simulink model "MotorCtrl_FOC_Math"  (R2025b)
settings: Solver=FixedStepDiscrete  StartTime=0.0  StopTime=5  FixedStep=MC_Sim_BaseStep  RelTol=1e-3  EnableMultiTasking=on
values from neighbouring files (symbols this model uses):
  MC_ADC_BitNum = 0.0    [MotorControlDataDictionary_Math.sldd]
  MC_ADC_Offset = 0.0    [MotorControlDataDictionary_Math.sldd]
  MC_ADC_VRef = 1.0    [MotorControlDataDictionary_Math.sldd]
  MC_CSA_Gain = 1.0    [MotorControlDataDictionary_Math.sldd]
  MC_MOS_DeadTime = 1.3E-6    [MotorControlDataDictionary_Math.sldd]
  MC_Motor_Mechinal_Damp = 1.0E-5    [MotorControlDataDictionary_Math.sldd]
  MC_Motor_Mechinal_Fric = 0.0    [MotorControlDataDictionary_Math.sldd]
  MC_Motor_Mechinal_Inertia = 0.0103    [MotorControlDataDictionary_Math.sldd]
  MC_Motor_Phi = 0.0059190254913385806    [MotorControlDataDictionary_Math.sldd]
  MC_Motor_Rotor_Pn = 4.0    [MotorControlDataDictionary_Math.sldd]
  MC_Motor_Stator_Ld = 5.6345E-5    [MotorControlDataDictionary_Math.sldd]
  MC_Motor_Stator_Lq = 5.6345E-5    [MotorControlDataDictionary_Math.sldd]
  MC_Motor_Stator_Rs = 0.0286    [MotorControlDataDictionary_Math.sldd]
  MC_Param_CurrentPI_Ki = 0.0089705790612839825    [MotorControlDataDictionary_Math.sldd]
  MC_Param_CurrentPI_Kp = 0.283220860906427    [MotorControlDataDictionary_Math.sldd]
  MC_Param_CurrentPI_UdInteMax = 7.794228634059948    [MotorControlDataDictionary_Math.sldd]
  MC_Param_CurrentPI_UdInteMin = -7.794228634059948    [MotorControlDataDictionary_Math.sldd]
  MC_Param_CurrentPI_UdMax = 7.794228634059948    [MotorControlDataDictionary_Math.sldd]
  MC_Param_CurrentPI_UdMin = -7.794228634059948    [MotorControlDataDictionary_Math.sldd]
  MC_Param_CurrentPI_UqInteMax = 7.794228634059948    [MotorControlDataDictionary_Math.sldd]
  MC_Param_CurrentPI_UqInteMin = -7.794228634059948    [MotorControlDataDictionary_Math.sldd]
  MC_Param_CurrentPI_UqMax = 7.794228634059948    [MotorControlDataDictionary_Math.sldd]
  MC_Param_CurrentPI_UqMin = -7.794228634059948    [MotorControlDataDictionary_Math.sldd]
  MC_Param_Flux_Gamma = 750000.0    [MotorControlDataDictionary_Math.sldd]
  MC_Param_Flux_Lalpha = 5.6345E-5    [MotorControlDataDictionary_Math.sldd]
  MC_Param_Flux_Lbeta = 5.6345E-5    [MotorControlDataDictionary_Math.sldd]
  MC_Param_Flux_Ralpha = 0.0286    [MotorControlDataDictionary_Math.sldd]
  MC_Param_Flux_Rbeta = 0.0286    [MotorControlDataDictionary_Math.sldd]
  MC_Param_Luen_BEMFalpha = -17747.803709290976    [MotorControlDataDictionary_Math.sldd]
  MC_Param_Luen_BEMFbeta = -17747.803709290976    [MotorControlDataDictionary_Math.sldd]
  MC_Param_Luen_BEMFErr = 10.0    [MotorControlDataDictionary_Math.sldd]
  MC_Param_Luen_Currentalpha = -507.58718608572195    [MotorControlDataDictionary_Math.sldd]
  MC_Param_Luen_Currentbeta = -507.58718608572195    [MotorControlDataDictionary_Math.sldd]
  MC_Param_Luen_CurrentErr = 400.0    [MotorControlDataDictionary_Math.sldd]
  MC_Param_Luen_PLL_Ki = 0.24634532585119037    [MotorControlDataDictionary_Math.sldd]
  MC_Param_Luen_PLL_Kp = 125.66370614359172    [MotorControlDataDictionary_Math.sldd]
  MC_Param_Luen_Voltagealpha = 17747.803709290976    [MotorControlDataDictionary_Math.sldd]
  MC_Param_Luen_Voltagebeta = 17747.803709290976    [MotorControlDataDictionary_Math.sldd]
  MC_Param_PhasetoReal = 500.0    [MotorControlDataDictionary_Math.sldd]
  MC_Param_SMO_CoffA = 0.968326559588251    [MotorControlDataDictionary_Math.sldd]
  MC_Param_SMO_CoffB = 1.1074629514597569    [MotorControlDataDictionary_Math.sldd]
  MC_Param_SpeedCtrl_IdMax = 60.0    [MotorControlDataDictionary_Math.sldd]
  MC_Param_SpeedCtrl_IdMin = -60.0    [MotorControlDataDictionary_Math.sldd]
  MC_Param_SpeedCtrl_IqMax = 60.0    [MotorControlDataDictionary_Math.sldd]
  MC_Param_SpeedCtrl_IqMin = -60.0    [MotorControlDataDictionary_Math.sldd]
  MC_Param_SpeedPI_Ki = 0.57157085739428382    [MotorControlDataDictionary_Math.sldd]
  MC_Param_SpeedPI_Kp = 9.1114109857344836    [MotorControlDataDictionary_Math.sldd]
  MC_Param_SpeedtoTheta = 6.24E-5    [MotorControlDataDictionary_Math.sldd]
  MC_Param_SVPWM_DutyMax = 0.98    [MotorControlDataDictionary_Math.sldd]
  MC_Param_SVPWM_DutyMin = 0.02    [MotorControlDataDictionary_Math.sldd]
  MC_Param_SVPWM_SampleOffset1 = 0.02    [MotorControlDataDictionary_Math.sldd]
  MC_Param_SVPWM_SampleOffset2 = 0.015    [MotorControlDataDictionary_Math.sldd]
  MC_Param_SVPWM_SampleValid = 0.0096153846153846159    [MotorControlDataDictionary_Math.sldd]
  MC_Param_Zero = 0.0    [MotorControlDataDictionary_Math.sldd]
  MC_Sample_CurrentNoise = 1.0E-15    [MotorControlDataDictionary_Math.sldd]
  MC_Sample_Rs = 0.002    [MotorControlDataDictionary_Math.sldd]
  MC_Sample_VbusNoise = 1.0E-15    [MotorControlDataDictionary_Math.sldd]
  MC_Sim_BaseStep = 2.08E-8    [MotorControlDataDictionary_Math.sldd]
  MC_Sim_HFTStep = 6.24E-5    [MotorControlDataDictionary_Math.sldd]
  MC_Sim_MFTStep = 0.0019968    [MotorControlDataDictionary_Math.sldd]
libraries: simulink x28, nesl_utility x19, fl_lib x14, ee_lib x13, autolibpmsminterior x2, autolibinverter x1
(part 4 of 8)

== system MotorCtrl_FOC_Math/MFTask/adrcofSpeed ==
  SpeedTarget : Inport
  SpeedReal : Inport  Port=2
  Constant : Constant  Value=0  OutDataTypeStr=single
  Delay One Step : Delay  DelayLength=1  InitialCondition=MC_Param_Zero
  ESO : Subsystem
  LESO : Subsystem  VariantControl=ESO
  NLSEF : Subsystem
  Tracking-Differentiator : Subsystem  Commented=on
  IdRef : Outport
  IqRef : Outport  Port=2
  wires:
  SpeedTarget/1 -> NLSEF/1(" SpeedRef"), Tracking-Differentiator/1(Ref_In)
  NLSEF/1(IqRef) -> IqRef/1, Delay One Step/1
  Tracking-Differentiator/1(SpeedTarget_TD) -> ?
  Delay One Step/1 -> ESO/2(u)
  ESO/1(z1) -> NLSEF/2(" z")
  ESO/2(z2) -> NLSEF/3(" d")
  Constant/1 -> IdRef/1
  SpeedReal/1 -> ESO/1(SpeedReal)

== system MotorCtrl_FOC_Math/MFTask/getCurrentLimit ==
  IdRef : Inport
  IqRef : Inport  Port=2
  Saturation : Saturate  UpperLimit=MC_Param_SpeedCtrl_IqMax  LowerLimit=MC_Param_SpeedCtrl_IqMin
  Saturation1 : Saturate  UpperLimit=MC_Param_SpeedCtrl_IdMax  LowerLimit=MC_Param_SpeedCtrl_IdMin
  Signal Copy : SignalConversion  OverrideOpt=off
  Signal Copy1 : SignalConversion  OverrideOpt=off
  IdRefLimit : Outport
  IqRefLimit : Outport  Port=2
  wires:
  IqRef/1 -> Saturation/1
  IdRef/1 -> Saturation1/1
  Signal Copy/1 -> IdRefLimit/1  "IdRefLimit"
  Signal Copy1/1 -> IqRefLimit/1  "IqRefLimit"
  Saturation/1 -> Signal Copy1/1
  Saturation1/1 -> Signal Copy/1

== system MotorCtrl_FOC_Math/MFTask/piofSpeed ==
  SpeedTarget : Inport
  SpeedReal : Inport  Port=2
  Abs : Abs  SaturateOnIntegerOverflow=off
  Add : Sum
  Add1 : Sum
  Compare To Constant : simulink/Logic and Bit Operations/Compare To Constant  relop=>  const=0.01  OutDataTypeStr=boolean
  Constant : Constant  Value=0  OutDataTypeStr=single
  Constant1 : Constant  Value=0  OutDataTypeStr=single
  Delay One Step : Delay  DelayLength=1
  Gain : Gain  Gain=MC_Param_SpeedPI_Kp
  Gain1 : Gain  Gain=MC_Param_SpeedPI_Ki
  Saturation : Saturate  UpperLimit=50  LowerLimit=-50
  Saturation1 : Saturate  UpperLimit=50  LowerLimit=-50
  Subtract : Sum  Inputs=+-
  Switch : Switch  Criteria=u2 > Threshold  SaturateOnIntegerOverflow=off  InputSameDT=off
  IdRef : Outport
  IqRef : Outport  Port=2
  wires:
  Add/1 -> Saturation/1, Delay One Step/1
  Subtract/1 -> Switch/1, Abs/1, Gain/1
  Gain1/1 -> Add/1
  Saturation/1 -> Add1/2
  Delay One Step/1 -> Add/2
  Gain/1 -> Add1/1
  Compare To Constant/1 -> Switch/2
  Add1/1 -> Saturation1/1
  Abs/1 -> Compare To Constant/1
  Constant/1 -> Switch/3
  SpeedReal/1 -> Subtract/2
  SpeedTarget/1 -> Subtract/1
  Switch/1 -> Gain1/1
  Constant1/1 -> IdRef/1  "IdRef"
  Saturation1/1 -> IqRef/1  "IqRef"

== system MotorCtrl_FOC_Math/MFTask/smcofSpeed ==
  note: 滑模控制：
      | 构建状态变量
  SpeedTarget : Inport
  SpeedReal : Inport  Port=2
  Add : Sum
  Add1 : Sum
  Add2 : Sum
  Constant : Constant  Value=0  OutDataTypeStr=single
  Delay One Step : Delay  DelayLength=1
  Delay One Step1 : Delay  DelayLength=1
  Gain : Gain  Gain=1/MC_Sim_MFTStep
  Gain1 : Gain  Gain=200
  Gain2 : Gain  Gain=50
  Gain3 : Gain  Gain=MC_Sim_MFTStep*1*MC_Motor_Mechinal_Inertia/(3*MC_Motor_Phi*MC_Motor_Rotor_Pn)
  Saturation : Saturate  UpperLimit=2  LowerLimit=-2
  Subtract : Sum  Inputs=+-
  Subtract1 : Sum  Inputs=+-
  IdRef : Outport
  IqRef : Outport  Port=2
  wires:
  SpeedTarget/1 -> Subtract/1
  SpeedReal/1 -> Subtract/2
  Subtract/1 -> Delay One Step/1, Subtract1/1, Add/1  "E1"
  Delay One Step/1 -> Subtract1/2
  Subtract1/1 -> Gain/1
  Gain/1 -> Add/2, Gain2/1  "E2"
  Add/1 -> Saturation/1  "S"
  Saturation/1 -> Gain1/1  "sign(S)"
  Gain1/1 -> Add1/1
  Gain2/1 -> Add1/2
  Add1/1 -> Gain3/1  "IqRef_dot"
  Gain3/1 -> Add2/1
  Add2/1 -> IqRef/1, Delay One Step1/1  "IqRef"
  Delay One Step1/1 -> Add2/2
  Constant/1 -> IdRef/1  "IdRef"

== system MotorCtrl_FOC_Math/Tracking-Differentiator/fastFunc1_TD ==
  Ref_In : Inport
  X1 : Inport  Port=2
  X2 : Inport  Port=3
  Abs1 : Abs  SaturateOnIntegerOverflow=off
  Add : Sum
  Add1 : Sum
  Add2 : Sum
  Constant : Constant  Value=0.01  OutDataTypeStr=single
  Gain : Gain  Gain=MC_Sim_MFTStep  ParamDataTypeStr=single  OutDataTypeStr=single  RndMeth=Simplest
  Gain1 : Gain  Gain=MC_Sim_MFTStep  ParamDataTypeStr=single  OutDataTypeStr=single  RndMeth=Simplest
  Gain2 : Gain  Gain=MC_Sim_MFTStep  ParamDataTypeStr=single  OutDataTypeStr=single  RndMeth=Simplest
  Gain3 : Gain  Gain=8  ParamDataTypeStr=single  OutDataTypeStr=single  RndMeth=Simplest
  Gain4 : Gain  Gain=1/2  ParamDataTypeStr=single  OutDataTypeStr=single  RndMeth=Simplest
  Gain5 : Gain  Gain=1/MC_Sim_MFTStep  ParamDataTypeStr=single  OutDataTypeStr=single  RndMeth=Simplest
  Gain6 : Gain  Commented=on
  Gain7 : Gain  Gain=1/MC_Sim_MFTStep  ParamDataTypeStr=single  OutDataTypeStr=single  RndMeth=Simplest
  Gain8 : Gain  Gain=-1  ParamDataTypeStr=single  OutDataTypeStr=single  RndMeth=Simplest
  Product : Product  OutDataTypeStr=single  RndMeth=Simplest
  Product1 : Product
  Product2 : Product  Commented=on
  Relational Operator : RelationalOperator  Operator=>  OutDataTypeStr=boolean  RndMeth=Simplest  InputSameDT=off
  Relational Operator1 : RelationalOperator  Operator=<=  OutDataTypeStr=boolean  RndMeth=Simplest  InputSameDT=off
  Sign : Signum
  Sign1 : Signum  Commented=on
  Sqrt : Sqrt
  Square : Math  Operator=square
  Subtract : Sum  Inputs=+-
  Subtract1 : Sum  Inputs=+-
  Switch : Switch  Criteria=u2 > Threshold  OutDataTypeStr=single  RndMeth=Simplest  SaturateOnIntegerOverflow=off  InputSameDT=off
  Switch1 : Switch  Criteria=u2 > Threshold  OutDataTypeStr=single  RndMeth=Simplest  SaturateOnIntegerOverflow=off  InputSameDT=off
  Ref_TD : Outport
  wires:
  X2/1 -> [x2]
  Ref_In/1 -> [Ref_In]
  X1/1 -> [x1]
  [x2] -> Gain/1
  Gain/1 -> Add/2
  [e] -> Add/1
  Add/1 -> [y]  "y"
  Subtract/1 -> [e]  "e"
  Constant/1 -> Gain3/1, Product1/2, Gain1/1  "r"
  Gain1/1 -> Gain2/1, [d]  "d"
  Gain2/1 -> [d0]  "d0"
  [y] -> Relational Operator/1, Sign1/1, Product/2
  Gain3/1 -> Product/1
  [d] -> Subtract1/2, Square/1
  Product/1 -> Add1/1
  Square/1 -> Add1/2
  Add1/1 -> Sqrt/1
  [d0] -> Relational Operator/2
  Relational Operator/1 -> Switch/2  "y_d0_Comp"
  Switch/1 -> Add2/1
  [x2] -> Add2/2
  [a0] -> Subtract1/1
  Subtract1/1 -> Gain4/1
  Gain4/1 -> Switch/1  "(a0-d)/2"
  [y] -> Gain5/1
  Gain5/1 -> Switch/3  "y/h"
  Add2/1 -> [a]  "a"
  Abs1/1 -> Relational Operator1/1
  [d] -> Relational Operator1/2
  Relational Operator1/1 -> Switch1/2  "a_d_Comp"
  Switch1/1 -> Gain8/1  "Ref_TD"
  [a] -> Gain7/1, Sign/1, Abs1/1
  Gain7/1 -> Switch1/1  "ra/d"
  Sign/1 -> Product1/1
  Product1/1 -> Switch1/3  "rsign(a)"
  Gain8/1 -> Ref_TD/1  "N_Ref_TD"
  [x1] -> Subtract/1
  [Ref_In] -> Subtract/2
  Sign1/1 -> Gain6/1
  Sqrt/1 -> [a0], Product2/1  "a0"
  Gain6/1 -> Product2/2

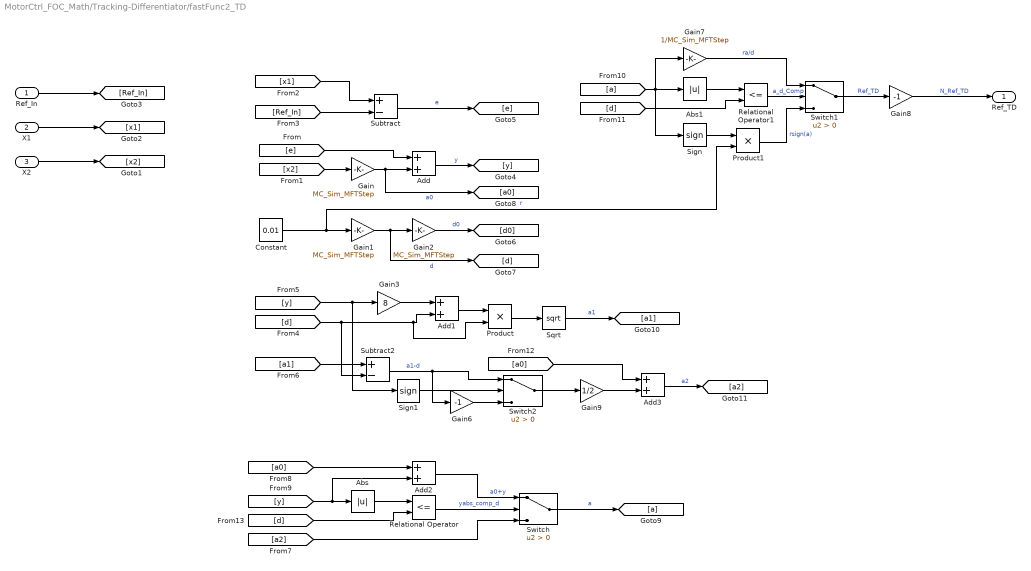
== system MotorCtrl_FOC_Math/Tracking-Differentiator/fastFunc2_TD ==
  Ref_In : Inport
  X1 : Inport  Port=2
  X2 : Inport  Port=3
  Abs : Abs  SaturateOnIntegerOverflow=off
  Abs1 : Abs  SaturateOnIntegerOverflow=off
  Add{,1..3} (4 alike) : Sum
  Constant : Constant  Value=0.01  OutDataTypeStr=single
  Gain : Gain  Gain=MC_Sim_MFTStep  ParamDataTypeStr=single  OutDataTypeStr=single  RndMeth=Simplest
  Gain1 : Gain  Gain=MC_Sim_MFTStep  ParamDataTypeStr=single  OutDataTypeStr=single  RndMeth=Simplest
  Gain2 : Gain  Gain=MC_Sim_MFTStep  ParamDataTypeStr=single  OutDataTypeStr=single  RndMeth=Simplest
  Gain3 : Gain  Gain=8
  Gain6 : Gain  Gain=-1  ParamDataTypeStr=single  OutDataTypeStr=single  RndMeth=Simplest
  Gain7 : Gain  Gain=1/MC_Sim_MFTStep  ParamDataTypeStr=single  OutDataTypeStr=single  RndMeth=Simplest
  Gain8 : Gain  Gain=-1  ParamDataTypeStr=single  OutDataTypeStr=single  RndMeth=Simplest
  Gain9 : Gain  Gain=1/2  ParamDataTypeStr=single  OutDataTypeStr=single  RndMeth=Simplest
  Product : Product
  Product1 : Product
  Relational Operator : RelationalOperator  Operator=<=  OutDataTypeStr=boolean  RndMeth=Simplest  InputSameDT=off
  Relational Operator1 : RelationalOperator  Operator=<=  OutDataTypeStr=boolean  RndMeth=Simplest  InputSameDT=off
  Sign : Signum
  Sign1 : Signum
  Sqrt : Sqrt
  Subtract : Sum  Inputs=+-
  Subtract2 : Sum  Inputs=+-  OutDataTypeStr=single  RndMeth=Simplest
  Switch : Switch  Criteria=u2 > Threshold  OutDataTypeStr=single  RndMeth=Simplest  SaturateOnIntegerOverflow=off  InputSameDT=off
  Switch1 : Switch  Criteria=u2 > Threshold  OutDataTypeStr=single  RndMeth=Simplest  SaturateOnIntegerOverflow=off  InputSameDT=off
  Switch2 : Switch  Criteria=u2 > Threshold  OutDataTypeStr=single  RndMeth=Simplest  SaturateOnIntegerOverflow=off  InputSameDT=off
  Ref_TD : Outport
  wires:
  [Ref_In] -> Subtract/2
  [x1] -> Subtract/1
  Gain8/1 -> Ref_TD/1  "N_Ref_TD"
  Product1/1 -> Switch1/3  "rsign(a)"
  Sign/1 -> Product1/1
  Gain7/1 -> Switch1/1  "ra/d"
  [a] -> Abs1/1, Sign/1, Gain7/1
  Switch1/1 -> Gain8/1  "Ref_TD"
  Relational Operator1/1 -> Switch1/2  "a_d_Comp"
  [d] -> Relational Operator1/2
  Abs1/1 -> Relational Operator1/1
  Gain3/1 -> Add1/1
  [d] -> Subtract2/2, Add1/2, Product/2
  Gain2/1 -> [d0]  "d0"
  Gain1/1 -> [d], Gain2/1  "d"
  Constant/1 -> Product1/2, Gain1/1  "r"
  Subtract/1 -> [e]  "e"
  Add/1 -> [y]  "y"
  [e] -> Add/1
  Gain/1 -> [a0], Add/2  "a0"
  [x2] -> Gain/1
  X1/1 -> [x1]
  Ref_In/1 -> [Ref_In]
  X2/1 -> [x2]
  [y] -> Sign1/1, Gain3/1
  Add1/1 -> Product/1
  Product/1 -> Sqrt/1
  Sqrt/1 -> [a1]  "a1"
  Sign1/1 -> Switch2/2
  [a1] -> Subtract2/1
  Subtract2/1 -> Gain6/1, Switch2/1  "a1-d"
  Gain6/1 -> Switch2/3
  Switch2/1 -> Gain9/1
  Gain9/1 -> Add3/2
  [a0] -> Add3/1
  Add3/1 -> [a2]  "a2"
  [y] -> Add2/2, Abs/1
  Abs/1 -> Relational Operator/1
  Relational Operator/1 -> Switch/2  "yabs_comp_d"
  [d] -> Relational Operator/2
  [a0] -> Add2/1
  Add2/1 -> Switch/1  "a0+y"
  [a2] -> Switch/3
  Switch/1 -> [a]  "a"

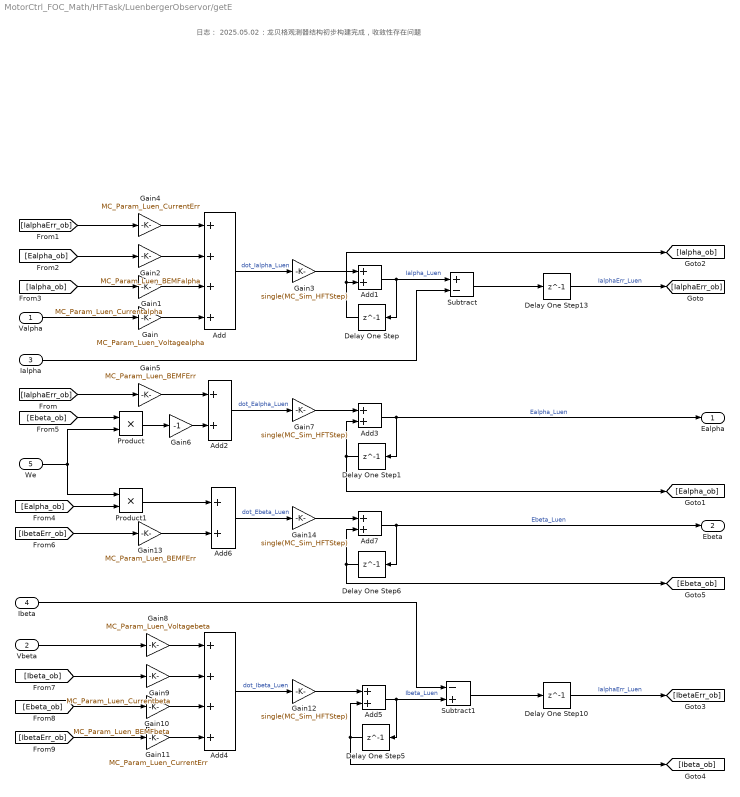
== system MotorCtrl_FOC_Math/HFTask/LuenbergerObservor/getE ==
  note: 日志：
      | 2025.05.02：龙贝格观测器结构初步构建完成，收敛性存在问题
  Valpha : Inport
  Vbeta : Inport  Port=2
  Ialpha : Inport  Port=3
  Ibeta : Inport  Port=4
  We : Inport  Port=5
  Add : Sum  Inputs=++++
  Add{1..3,5..7} (6 alike) : Sum
  Add4 : Sum  Inputs=++++
  Delay One Step{,1,5..6,10,13} (6 alike) : Delay  DelayLength=1
  Gain : Gain  Gain=MC_Param_Luen_Voltagealpha
  Gain1 : Gain  Gain=MC_Param_Luen_Currentalpha
  Gain10 : Gain  Gain=MC_Param_Luen_BEMFbeta
  Gain11 : Gain  Gain=MC_Param_Luen_CurrentErr
  Gain{3,7,12,14} (4 alike) : Gain  Gain=single(MC_Sim_HFTStep)
  Gain13 : Gain  Gain=MC_Param_Luen_BEMFErr
  Gain2 : Gain  Gain=MC_Param_Luen_BEMFalpha
  Gain4 : Gain  Gain=MC_Param_Luen_CurrentErr
  Gain5 : Gain  Gain=MC_Param_Luen_BEMFErr
  Gain6 : Gain  Gain=-1
  Gain8 : Gain  Gain=MC_Param_Luen_Voltagebeta
  Gain9 : Gain  Gain=MC_Param_Luen_Currentbeta
  Product : Product
  Product1 : Product
  Subtract : Sum  Inputs=+-
  Subtract1 : Sum  Inputs=-+
  Ealpha : Outport
  Ebeta : Outport  Port=2
  wires:
  Valpha/1 -> Gain/1
  Add/1 -> Gain3/1  "dot_Ialpha_Luen"
  Gain2/1 -> Add/2
  Gain1/1 -> Add/3
  Gain/1 -> Add/4
  Gain4/1 -> Add/1
  Gain3/1 -> Add1/1
  Add1/1 -> Subtract/1, Delay One Step/1  "Ialpha_Luen"
  Delay One Step/1 -> [Ialpha_ob], Add1/2
  Ialpha/1 -> Subtract/2
  Subtract/1 -> Delay One Step13/1
  [IalphaErr_ob] -> Gain5/1
  Gain5/1 -> Add2/1
  Gain6/1 -> Add2/2
  Add2/1 -> Gain7/1  "dot_Ealpha_Luen"
  Delay One Step1/1 -> Add3/2, [Ealpha_ob]
  Add3/1 -> Ealpha/1, Delay One Step1/1  "Ealpha_Luen"
  Gain7/1 -> Add3/1
  Product/1 -> Gain6/1
  We/1 -> Product/2, Product1/1
  Vbeta/1 -> Gain8/1
  Gain8/1 -> Add4/1
  Gain9/1 -> Add4/2
  Gain10/1 -> Add4/3
  Gain11/1 -> Add4/4
  [IalphaErr_ob] -> Gain4/1
  [Ealpha_ob] -> Gain2/1
  [Ialpha_ob] -> Gain1/1
  Add4/1 -> Gain12/1  "dot_Ibeta_Luen"
  Delay One Step5/1 -> Add5/2, [Ibeta_ob]
  Add5/1 -> Subtract1/2, Delay One Step5/1  "Ibeta_Luen"
  Gain12/1 -> Add5/1
  Ibeta/1 -> Subtract1/1
  Subtract1/1 -> Delay One Step10/1
  Add6/1 -> Gain14/1  "dot_Ebeta_Luen"
  Gain13/1 -> Add6/2
  Product1/1 -> Add6/1
  Gain14/1 -> Add7/1
  Add7/1 -> Ebeta/1, Delay One Step6/1  "Ebeta_Luen"
  Delay One Step6/1 -> Add7/2, [Ebeta_ob]
  [Ealpha_ob] -> Product1/2
  [Ebeta_ob] -> Product/1
  [IbetaErr_ob] -> Gain13/1
  [Ibeta_ob] -> Gain9/1
  [IbetaErr_ob] -> Gain11/1
  [Ebeta_ob] -> Gain10/1
  Delay One Step13/1 -> [IalphaErr_ob]  "IalphaErr_Luen"
  Delay One Step10/1 -> [IbetaErr_ob]  "IalphaErr_Luen"

== system MotorCtrl_FOC_Math/HFTask/LuenbergerObservor/getSpeedandTheta ==
  note: 日志：
      | 2025.03.19：反电势正负号识别错误，改正后可以使用
  Ealpha : Inport
  Ebeta : Inport  Port=2
  Add : Sum
  Add1 : Sum
  Add2 : Sum
  Constant : Constant  Value=2*pi  OutDataTypeStr=single
  Delay One Step : Delay  DelayLength=1
  Delay One Step2 : Delay  DelayLength=1
  Gain1 : Gain  Gain=MC_Param_Luen_PLL_Kp
  Gain2 : Gain  Gain=MC_Param_Luen_PLL_Ki
  Gain3 : Gain  Gain=MC_Param_SpeedtoTheta
  Gain5 : Gain  Gain=30/(pi*MC_Motor_Rotor_Pn)  OutDataTypeStr=single  RndMeth=Simplest
  Mod : Math  Operator=mod
  Product : Product
  Product1 : Product
  Sin : Trigonometry  OutputSignalType=real
  Sin1 : Trigonometry  Operator=cos  OutputSignalType=real
  Subtract : Sum  Inputs=+-
  Speed : Outport
  Theta : Outport  Port=2
  We : Outport  Port=3
  wires:
  Gain5/1 -> Speed/1  "SpeedLuen_RPM"
  Product1/1 -> Subtract/2  "LuenCos"
  Product/1 -> Subtract/1  "LuenSin"
  [Theta_Last] -> Sin/1, Sin1/1
  Add1/1 -> We/1, Gain3/1, Gain5/1  "WeLuen"
  Mod/1 -> Delay One Step2/1, Theta/1  "ThetaLuen"
  Delay One Step2/1 -> [Theta_Last], Add2/2
  Constant/1 -> Mod/2
  Add2/1 -> Mod/1
  Gain3/1 -> Add2/1
  Subtract/1 -> Gain1/1, Gain2/1  "LuenErr"
  Gain1/1 -> Add1/1
  Delay One Step/1 -> Add/2
  Add/1 -> Add1/2, Delay One Step/1
  Gain2/1 -> Add/1
  Sin/1 -> Product1/2
  Sin1/1 -> Product/2
  Ealpha/1 -> Product1/1
  Ebeta/1 -> Product/1

== system MotorCtrl_FOC_Math/HFTask/currentADRC/LESO ==
  Id : Inport
  Ud : Inport  Port=2
  Iq : Inport  Port=3
  Uq : Inport  Port=4
  Add1 : Sum  Inputs=+++  AccumDataTypeStr=single  RndMeth=Simplest
  Add{2,4..6} (4 alike) : Sum
  Add3 : Sum  Inputs=+++  AccumDataTypeStr=single  RndMeth=Simplest
  Delay{,1..3} (4 alike) : Delay  DelayLength=1  InitialCondition=single(0)
  Gain1 : Gain  Gain=2*pi*100*2*pi*100
  Gain2 : Gain  Gain=2*2*pi*100
  Gain4 : Gain  Gain=2*pi*100*2*pi*100
  Gain5 : Gain  Gain=2*2*pi*100
  Gain6 : Gain  Gain=1/single(MC_Motor_Stator_Ld)
  Gain7 : Gain  Gain=1/single(MC_Motor_Stator_Lq)
  Subtract1 : Sum  Inputs=+-
  Subtract2 : Sum  Inputs=+-
  Ts{1..4} (4 alike) : Gain  Gain=single(MC_Sim_HFTStep)  ParamDataTypeStr=single  OutDataTypeStr=single  RndMeth=Simplest
  falFunc : Subsystem  Commented=on
  Id_ESO : Outport
  Iq_ESO : Outport  Port=2
  Id_Dis : Outport  Port=3
  Iq_Dis : Outport  Port=4
  wires:
  [Id_ESO_Delay] -> Subtract1/2
  Id/1 -> Subtract1/1
  Gain2/1 -> Add3/2
  Ud/1 -> Gain6/1
  Add3/1 -> Ts1/1
  Ts1/1 -> Add4/1
  Add4/1 -> Delay/1, Id_ESO/1  "Id_ESO"
  Delay/1 -> Add4/2, [Id_ESO_Delay]
  Subtract1/1 -> Gain1/1, Gain2/1
  Add5/1 -> Id_Dis/1, Delay1/1  "Id_Dis"
  Gain1/1 -> Ts2/1
  Ts2/1 -> Add5/1
  Delay1/1 -> Add3/3, Add5/2
  Delay3/1 -> Add1/3, Add6/2
  Ts4/1 -> Add6/1
  Gain4/1 -> Ts4/1
  Add6/1 -> Iq_Dis/1, Delay3/1  "Iq_Dis"
  Subtract2/1 -> Gain4/1, Gain5/1
  Delay2/1 -> [Iq_ESO_Delay], Add2/2
  Add2/1 -> Iq_ESO/1, Delay2/1  "Iq_ESO"
  Ts3/1 -> Add2/1
  Add1/1 -> Ts3/1
  Uq/1 -> Gain7/1
  Gain5/1 -> Add1/2
  Iq/1 -> Subtract2/1
  [Iq_ESO_Delay] -> Subtract2/2
  Gain6/1 -> Add3/1  "bUd"
  Gain7/1 -> Add1/1  "bUq"

== system MotorCtrl_FOC_Math/HFTask/currentADRC/NLSEF ==
  Id_Ref : Inport
  Iq_Ref : Inport  Port=2
  Id_ESO : Inport  Port=3
  Iq_ESO : Inport  Port=4
  Id_ESO_Dis : Inport  Port=5
  Iq_ESO_Dis : Inport  Port=6
  Gain1 : Gain  Gain=0.1  OutDataTypeStr=single  RndMeth=Simplest
  Gain2 : Gain  Gain=0.1  OutDataTypeStr=single  RndMeth=Simplest
  Gain3 : Gain  Gain=single(MC_Motor_Stator_Ld)  OutDataTypeStr=single  RndMeth=Simplest
  Gain5 : Gain  Gain=single(MC_Motor_Stator_Lq)  OutDataTypeStr=single  RndMeth=Simplest
  Saturation : Saturate  UpperLimit=MC_Param_CurrentPI_UdMax  LowerLimit=MC_Param_CurrentPI_UdMin
  Saturation1 : Saturate  UpperLimit=MC_Param_CurrentPI_UqMax  LowerLimit=MC_Param_CurrentPI_UqMin
  Subtract : Sum  Inputs=+-
  Subtract1 : Sum  Inputs=+-  OutDataTypeStr=single  AccumDataTypeStr=single  RndMeth=Simplest
  Subtract2 : Sum  Inputs=+-
  Subtract3 : Sum  Inputs=+-
  Ud_ADRC : Outport
  Uq_ADRC : Outport  Port=2
  wires:
  Id_Ref/1 -> Subtract/1
  Id_ESO/1 -> Subtract/2
  Subtract2/1 -> Saturation/1  "Ud_ADRC"
  Saturation/1 -> Ud_ADRC/1
  Saturation1/1 -> Uq_ADRC/1
  Subtract3/1 -> Saturation1/1  "Uq_ADRC"
  Iq_ESO/1 -> Subtract1/2
  Iq_Ref/1 -> Subtract1/1
  Id_ESO_Dis/1 -> Gain3/1
  Gain3/1 -> Subtract2/2
  Iq_ESO_Dis/1 -> Gain5/1
  Gain5/1 -> Subtract3/2
  Gain2/1 -> Subtract3/1
  Subtract/1 -> Gain1/1  "Id_Err"
  Gain1/1 -> Subtract2/1
  Subtract1/1 -> Gain2/1  "Iq_Err"

== system MotorCtrl_FOC_Math/HFTask/currentPIRControl/currentRController_D ==
  CurrErr : Inport
  Wm : Inport  Port=2
  UReal : Inport  Port=3
  Add : Sum  Inputs=+---
  Delay One Step : Delay  DelayLength=1  InitialCondition=single(0)
  Delay One Step1 : Delay  InitialCondition=single(0)
  Delay One Step2 : Delay  InitialCondition=single(0)
  Gain{,1..3} (4 alike) : Gain
  Saturation : Saturate
  Terminator : Terminator
  Terminator1 : Terminator
  UR_Ref : Outport
  wires:
  Gain/1 -> Add/1
  CurrErr/1 -> Delay One Step2/1, Gain/1
  Delay One Step2/1 -> Gain1/1
  Gain1/1 -> Add/2
  Wm/1 -> Terminator/1
  UReal/1 -> Terminator1/1
  Add/1 -> Saturation/1
  Delay One Step/1 -> Gain2/1
  Delay One Step1/1 -> Gain3/1
  Gain3/1 -> Add/4
  Gain2/1 -> Add/3
  Saturation/1 -> Delay One Step/1, Delay One Step1/1, UR_Ref/1

== system MotorCtrl_FOC_Math/HFTask/currentPIRControl/currentRController_Q ==
  CurrErr : Inport
  Wm : Inport  Port=2
  UReal : Inport  Port=3
  Add : Sum  Inputs=+---
  Delay One Step : Delay  DelayLength=1  InitialCondition=single(0)
  Delay One Step1 : Delay  InitialCondition=single(0)
  Delay One Step2 : Delay  InitialCondition=single(0)
  Gain{,1..3} (4 alike) : Gain
  Saturation : Saturate
  Terminator : Terminator
  Terminator1 : Terminator
  UR_Ref : Outport
  wires:
  Saturation/1 -> UR_Ref/1, Delay One Step1/1, Delay One Step/1
  Gain2/1 -> Add/3
  Gain3/1 -> Add/4
  Delay One Step1/1 -> Gain3/1
  Delay One Step/1 -> Gain2/1
  Add/1 -> Saturation/1
  UReal/1 -> Terminator1/1
  Wm/1 -> Terminator/1
  Gain1/1 -> Add/2
  Delay One Step2/1 -> Gain1/1
  CurrErr/1 -> Gain/1, Delay One Step2/1
  Gain/1 -> Add/1

== system MotorCtrl_FOC_Math/HFTask/fluxobservor/getFlux ==
  note: 日志：
      | 2025.02.28：滑膜观测器建模无问题，但是反电势观测存在问题，暂时分析为参数问题
  Valpha : Inport
  Vbeta : Inport  Port=2
  Ialpha : Inport  Port=3
  Ibeta : Inport  Port=4
  Add{,1..4} (5 alike) : Sum
  Constant : Constant  Value=MC_Motor_Phi  OutDataTypeStr=single
  Delay One Step{,1..3} (4 alike) : Delay  DelayLength=1
  Gain : Gain  Gain=MC_Param_Flux_Ralpha
  Gain1 : Gain  Gain=MC_Param_Flux_Gamma  OutDataTypeStr=single  RndMeth=Simplest
  Gain2 : Gain  Gain=single(MC_Sim_HFTStep)  OutDataTypeStr=single  RndMeth=Simplest
  Gain3 : Gain  Gain=MC_Param_Flux_Lalpha  OutDataTypeStr=single  RndMeth=Simplest
  Gain4 : Gain  Gain=MC_Param_Flux_Rbeta
  Gain5 : Gain  Gain=MC_Param_Flux_Gamma  OutDataTypeStr=single  RndMeth=Simplest
  Gain6 : Gain  Gain=single(MC_Sim_HFTStep)
  Gain7 : Gain  Gain=MC_Param_Flux_Lbeta  OutDataTypeStr=single  RndMeth=Simplest
  Product : Product
  Product1 : Product
  Square : Math  Operator=square
  Square1 : Math  Operator=square
  Square2 : Math  Operator=square
  Subtract{,1..4} (5 alike) : Sum  Inputs=+-
  Phialpha : Outport
  Phibeta : Outport  Port=2
  wires:
  Valpha/1 -> Subtract/1
  Ialpha/1 -> Gain3/1, Gain/1
  Gain/1 -> Subtract/2
  Subtract/1 -> Add/1  "Y_Alpha"
  Gain1/1 -> Add/2  "NLFcn_Alpha"
  Add/1 -> Gain2/1  "Xdot_Alpha"
  Add1/1 -> Subtract1/1, Delay One Step/1  "X_Alpha"
  Delay One Step/1 -> Add1/2
  Gain2/1 -> Add1/1
  Gain3/1 -> Subtract1/2
  Subtract1/1 -> Phialpha/1, Delay One Step1/1  "Phialpha"
  Product/1 -> Gain1/1
  Delay One Step1/1 -> [Nx_alpha], Product/2
  Delay One Step3/1 -> [Nx_beta], Product1/2
  Product1/1 -> Gain5/1
  Subtract3/1 -> Phibeta/1, Delay One Step3/1  "Phibeta"
  Gain7/1 -> Subtract3/2
  Gain6/1 -> Add3/1
  Delay One Step2/1 -> Add3/2
  Add3/1 -> Delay One Step2/1, Subtract3/1  "X_Beta"
  Add2/1 -> Gain6/1  "Xdot_Beta"
  Gain5/1 -> Add2/2  "NLFcn_Beta"
  Subtract2/1 -> Add2/1  "Y_Beta"
  Gain4/1 -> Subtract2/2
  Ibeta/1 -> Gain4/1, Gain7/1
  Vbeta/1 -> Subtract2/1
  Constant/1 -> Square/1
  [Nx_alpha] -> Square1/1
  [Nx_beta] -> Square2/1
  Square1/1 -> Add4/1
  Square2/1 -> Add4/2
  Square/1 -> Subtract4/1
  Add4/1 -> Subtract4/2  "Psim2"
  Subtract4/1 -> [Nx2]  "Nx2"
  [Nx2] -> Product/1
  [Nx2] -> Product1/1

== system MotorCtrl_FOC_Math/HFTask/fluxobservor/getSpeedandTheta ==
  Phialpha : Inport
  Phibeta : Inport  Port=2
  Add : Sum
  Add1 : Sum
  Add2 : Sum
  Constant : Constant  Value=2*pi  OutDataTypeStr=single
  Delay One Step : Delay  DelayLength=1
  Delay One Step2 : Delay  DelayLength=1
  Gain : Gain  Gain=1/MC_Motor_Phi
  Gain1 : Gain  Gain=2*sqrt(2)/2*100
  Gain2 : Gain  Gain=100^2*MC_Sim_HFTStep
  Gain3 : Gain  Gain=MC_Param_SpeedtoTheta  OutDataTypeStr=single  RndMeth=Simplest
  Gain4 : Gain  Gain=1/MC_Motor_Phi
  Gain5 : Gain  Gain=30/(pi*MC_Motor_Rotor_Pn)  OutDataTypeStr=single  RndMeth=Simplest
  Mod : Math  Operator=mod
  Product : Product
  Product1 : Product
  Sin : Trigonometry  OutputSignalType=real
  Sin1 : Trigonometry  Operator=cos  OutputSignalType=real
  Subtract : Sum  Inputs=+-
  Speed : Outport
  Theta : Outport  Port=2
  wires:
  [Theta_Last] -> Sin/1, Sin1/1
  Add1/1 -> Gain5/1, Gain3/1  "WeFlux"
  Mod/1 -> Delay One Step2/1, Theta/1  "ThetaFlux"
  Delay One Step2/1 -> [Theta_Last], Add2/2
  Constant/1 -> Mod/2
  Add2/1 -> Mod/1
  Gain3/1 -> Add2/1
  Subtract/1 -> Gain1/1, Gain2/1  "FluxErr"
  Gain1/1 -> Add1/1
  Delay One Step/1 -> Add/2
  Add/1 -> Add1/2, Delay One Step/1
  Gain2/1 -> Add/1
  Product1/1 -> Subtract/2  "FluxSin"
  Product/1 -> Subtract/1  "FluxCos"
  Sin/1 -> Product1/2
  Sin1/1 -> Product/2
  Phibeta/1 -> Gain/1
  Phialpha/1 -> Gain4/1
  Gain/1 -> Product/1
  Gain4/1 -> Product1/1
  Gain5/1 -> Speed/1  "SpeedFlux_RPM"
